simulink model "Flight_Dynamics_Simulation"  (R2026a)
settings: Solver=ode45  StopTime=120
InitFcn:
  | %%% Sensor with 3D measurement
  | % Define elements
  | elems(1) = Simulink.BusElement;
  | elems(1).Name = 'meas';
  | elems(1).Dimensions = 3;
  | elems(1).DataType = 'double';
  | elems(2) = Simulink.BusElement;
  | elems(2).Name = 'status';
  | elems(2).Dimensions = 1;
  | elems(2).DataType = 'boolean';
  | % Create bus
  | Sensor3DBus = Simulink.Bus;
  | Sensor3DBus.Elements = elems;
  | 
  | %%% Sensor with 1D measurement
  | % Define elements
  | elems(1) = Simulink.BusElement;
  | elems(1).Name = 'meas';
  | elems(1).Dimensions = 1;
  | elems(1).DataType = 'double';
  | elems(2) = Simulink.BusElement;
  | elems(2).Name = 'status';
  | elems(2).Dimensions = 1;
  | elems(2).DataType = 'boolean';
  | % Create bus
  | Sensor1DBus = Simulink.Bus;
  | Sensor1DBus.Elements = elems;
undefined symbols (not defined in the file or in its folder): alt, angle_vert_deg, crossrange, location, sim_time, vel_ver
libraries: aerolibanim x2, sharedtransform x1, simulink_extras x1
settings Model: Creator=bruno  LastModifiedBy=trist
settings OptimizationCC: GainParamInheritBuiltInType=on  UseFloatMulNetSlope=on  InlineInvariantSignals=on  EfficientFloat2IntCast=on
settings DebuggingCC: ArrayBoundsChecking=warning  CheckMatrixSingularityMsg=warning  SFcnCompatibilityMsg=warning  UniqueDataStoreMsg=warning
settings HardwareCC: ProdBitPerLong=64.0  ProdHWDeviceType=AMD->x86-64 (Linux 64)
settings ModelReferenceCC: EnableParallelModelReferenceBuilds=on
settings SFSimCC: SimTargetLang=C++
settings RTWCC: Toolchain=Simulink Real-Time Linux x64 Remote Build Toolchain  BuildConfiguration=Faster Runs  TargetLang=C++  CheckMdlBeforeBuild=Warning
settings GRTTargetCC: TargetLangStandard=C++11 (ISO)  MatFileLogging=off  CodeInterfacePackaging=C++ class  SupportNonFinite=off

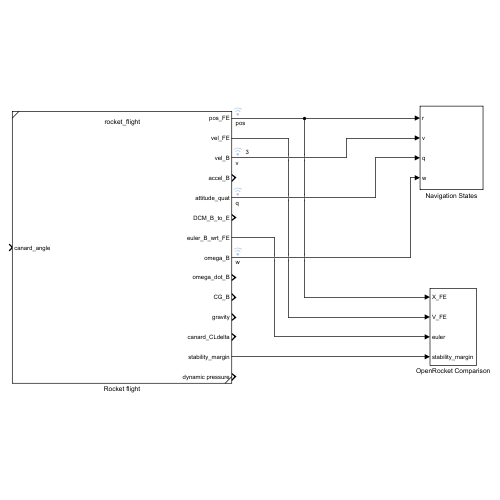
[thumbnail: Simulink's stored preview of the top-level diagram]
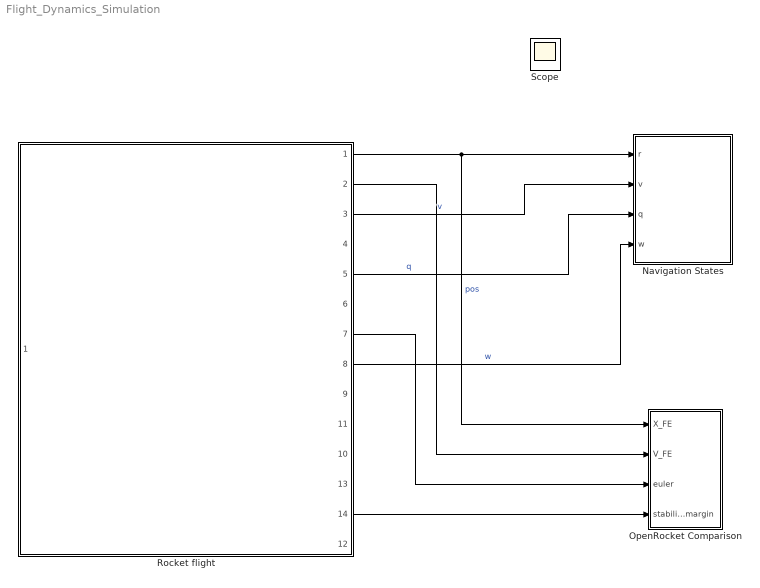
== system Flight_Dynamics_Simulation ==
  Navigation States : Subsystem
  OpenRocket Comparison : Subsystem
  Rocket flight : Subsystem  ReferencedSubsystem=rocket_flight
      settings: PortSchema="{\"entries\":[{\"content\":{\"sides\":[{\"content\":{\"connectorIds\":[\"In1\"]},\"type\":\"ConnectorPlacement.EquallySpacedRectSide\",\"uuid\":\"9f79cae0-15ae-41cc-86ca-52b2ba536b20\"},{\"content\":{\"connectorIds\":[\"Out1\",\"Out2\",\"Out3\",\"Out4\",\"Out5\",\"Out6\",\"Out7\",\"Out8\",\"Out9\",\"Out11\",\"Out10\",\"Out13\",\"Out14\",\"Out12\"],\"side\":\"RIGHT\"},\"type\":\"ConnectorPlacement.EquallySpacedRectSide\",\"uuid\":\"ebcb1700-a632-4dda-8ea5-5b87e6fa3b6a\"},{\"content\":{\"side\":\"TOP\"},\"type\":\"ConnectorPlacement.EquallySpacedRectSide\",\"uuid\":\"efdf61b2-36e8-47a1-89a6-5eee4bf93d92\"}]},\"type\":\"ConnectorPlacement.EquallySpacedConnector\",\"uuid\":\"49b511cd-3c57-4668-a103-5fb675f3d38c\"}],\"packageUris\":[\"http://schema.mathworks.com/mf0/Connector/R2020b\"],\"version\":\"1.0\"}"
  Scope : Scope
      settings: ActiveDisplayYMinimum=9.79326  ActiveDisplayYMaximum=9.80609
  wires:
  Rocket flight/1 -> Navigation States/4(r), OpenRocket Comparison/1(X_FE)  "pos"
  Rocket flight/8 -> Navigation States/1(w)  "w"
  Rocket flight/5 -> Navigation States/2(q)  "q"
  Rocket flight/3 -> Navigation States/3(v)  "v"
  Rocket flight/2 -> OpenRocket Comparison/2(V_FE)
  Rocket flight/7 -> OpenRocket Comparison/3(euler)
  Rocket flight/14 -> OpenRocket Comparison/4(stability_margin)

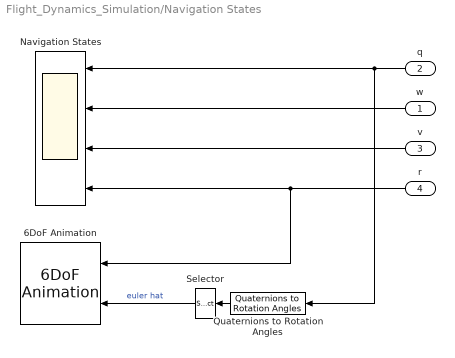
== system Flight_Dynamics_Simulation/Navigation States ==
  w : Inport
  q : Inport  Port=2
  v : Inport  Port=3
  r : Inport  Port=4
  6DoF Animation : aerolibanim/6DoF Animation  u1=[0 8000 -100 100 0 400]  u2=0.1  u3=5  u4=[location(1)-5 0 0]  u5=Fly alongside  u6=[0 100 0]  u7=10  u8=off
  Navigation States : Scope  NumInputPorts=4
      settings: Title=Attitude Quaternion  ActiveDisplayYMinimum=-1.2408627479450127  ActiveDisplayYMaximum=1.2486648107009546  DataLoggingVariableName=ScopeData7
  Quaternions to Rotation Angles : sharedtransform/Quaternions to Rotation Angles  rotationOrder=ZYX  aMode=aMode
  Selector : Selector  InputPortWidth=3  IndexOptions=Index vector (dialog)  Indices=[3 2 1]  OutputSizes=1
  wires:
  v/1 -> Navigation States/3
  Selector/1 -> 6DoF Animation/2  "euler hat"
  w/1 -> Navigation States/2
  q/1 -> Quaternions to Rotation Angles/1, Navigation States/1
  r/1 -> 6DoF Animation/1, Navigation States/4
  Quaternions to Rotation Angles/1 -> Selector/1

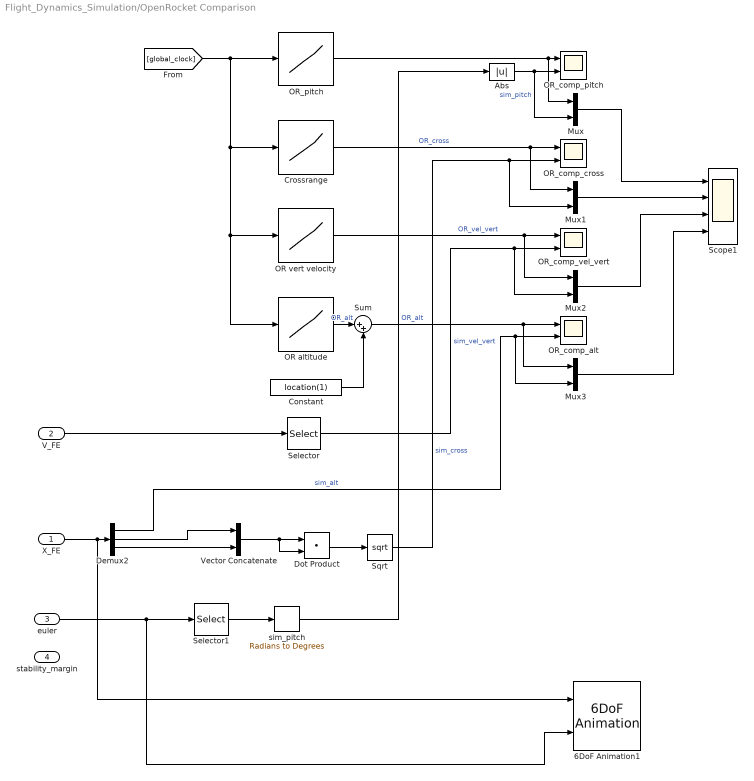
== system Flight_Dynamics_Simulation/OpenRocket Comparison ==
  X_FE : Inport
  V_FE : Inport  Port=2
  euler : Inport  Port=3
  stability_margin : Inport  Port=4
  6DoF Animation1 : aerolibanim/6DoF Animation  u1=[0 8000 -100 100 0 400]  u2=0.1  u3=5  u4=[location(1)-5 0 0]  u5=Fly alongside  u6=[-50 20 0]  u7=10  u8=off
  Abs : Abs  SaturateOnIntegerOverflow=off
  Constant : Constant  Value=location(1)
  Crossrange : Lookup_n-D  NumberOfTableDimensions=1  BreakpointsForDimension1=sim_time  Table=crossrange  InternalRulePriority=Speed  RndMeth=Simplest
  Demux2 : Demux  Outputs=3
  Dot Product : DotProduct  OutDataTypeStr=Inherit: Inherit via internal rule
  Mux{,1..3} (4 alike) : Mux  Inputs=2
  OR altitude : Lookup_n-D  NumberOfTableDimensions=1  BreakpointsForDimension1=sim_time  Table=alt  InternalRulePriority=Speed  RndMeth=Simplest
  OR vert velocity : Lookup_n-D  NumberOfTableDimensions=1  BreakpointsForDimension1=sim_time  Table=vel_ver  InternalRulePriority=Speed  RndMeth=Simplest
  OR_comp_alt : Scope  NumInputPorts=2
      settings: ActiveDisplayYMinimum=-838.88766  ActiveDisplayYMaximum=7549.94141  DataLoggingVariableName=ScopeData2
  OR_comp_cross : Scope  NumInputPorts=2
      settings: ActiveDisplayYMinimum=-199.36184  ActiveDisplayYMaximum=1794.25654  DataLoggingVariableName=ScopeData4
  OR_comp_pitch : Scope  NumInputPorts=2
      settings: ActiveDisplayYMinimum=-13.012  ActiveDisplayYMaximum=167.10802  DataLoggingVariableName=ScopeData8
  OR_comp_vel_vert : Scope  NumInputPorts=2
      settings: ActiveDisplayYMinimum=-95.80315  ActiveDisplayYMaximum=488.12758  DataLoggingVariableName=ScopeData10
  OR_pitch : Lookup_n-D  NumberOfTableDimensions=1  BreakpointsForDimension1=sim_time  Table=angle_vert_deg  InternalRulePriority=Speed  RndMeth=Simplest
  Scope1 : Scope  NumInputPorts=4
      settings: ActiveDisplayYMinimum=-5.57011622160341  ActiveDisplayYMaximum=50.131045994430721  DataLoggingVariableName=ScopeData11
  Selector : Selector  InputPortWidth=3  IndexOptions=Index vector (dialog)  Indices=[1]  OutputSizes=1
  Selector1 : Selector  InputPortWidth=3  IndexOptions=Index vector (dialog)  Indices=[2]  OutputSizes=1
  Sqrt : Sqrt
  Sum : Sum  Inputs=|++
  Vector Concatenate : Concatenate
  sim_pitch : simulink_extras/Transformations/Radians to Degrees
  wires:
  OR altitude/1 -> Sum/1  "OR_alt"
  Mux/1 -> Scope1/1
  [global_clock] -> Crossrange/1, OR vert velocity/1, OR altitude/1, OR_pitch/1
  OR vert velocity/1 -> Mux2/1, OR_comp_vel_vert/1  "OR_vel_vert"
  X_FE/1 -> 6DoF Animation1/1, Demux2/1
  Demux2/2 -> Vector Concatenate/1
  Abs/1 -> OR_comp_pitch/2, Mux/2  "sim_pitch"
  Demux2/1 -> Mux3/2, OR_comp_alt/2  "sim_alt"
  Sqrt/1 -> Mux1/2, OR_comp_cross/2  "sim_cross"
  Mux3/1 -> Scope1/4
  euler/1 -> 6DoF Animation1/2, Selector1/1
  Crossrange/1 -> OR_comp_cross/1, Mux1/1  "OR_cross"
  Sum/1 -> OR_comp_alt/1, Mux3/1  "OR_alt"
  OR_pitch/1 -> OR_comp_pitch/1, Mux/1
  Mux1/1 -> Scope1/2
  Selector/1 -> Mux2/2, OR_comp_vel_vert/2  "sim_vel_vert"
  Constant/1 -> Sum/2
  Dot Product/1 -> Sqrt/1
  V_FE/1 -> Selector/1
  Vector Concatenate/1 -> Dot Product/2, Dot Product/1
  Mux2/1 -> Scope1/3
  sim_pitch/1 -> Abs/1
  Selector1/1 -> sim_pitch/1
  Demux2/3 -> Vector Concatenate/2
